simulink model "Teste_ModeloPV"  (R2017a)
settings: Solver=VariableStepAuto  StartTime=0.0  StopTime=10.0  MinStep=0.1  RelTol=1e-3
libraries: simulink x3, AvgModels x1
settings Model: Creator=lgalotto  LastModifiedBy=lgalotto

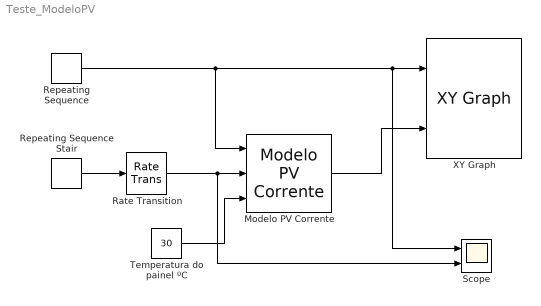
== system Teste_ModeloPV ==
  Modelo PV Corrente : AvgModels/Modelo PV Corrente  Ms=1  Mp=1  Ns=54  Voc=0.6093  Isc=8.21  Tr=273 + 25  Rs=0.005  Rp=7  a=3.18e-3  n=1.2  k=1.38e-23  q=1.60e-19  EG=1.1
      settings: SourceProductName=SimAverageModels
  Rate Transition : RateTransition  OutPortSampleTime=0.001
  Repeating Sequence : simulink/Sources/Repeating Sequence  rep_seq_t=[0 0.5 1]  rep_seq_y=[0 32 0]
  Repeating Sequence Stair : simulink/Sources/Repeating Sequence Stair  OutValues=[100 200 300 400 500 600 700 800 900 1000].'  tsamp=1  OutMin=[]  OutMax=[]  OutDataTypeStr=double  OutputDataTypeScalingMode=double  OutDataType=fixdt(0,8)  ConRadixGroup=Best Precision: Vector-wise  OutScaling=2^-12
  Scope : Scope  NumInputPorts=2
  Temperatura do painel ºC : Constant  Value=30
  XY Graph : simulink/Sinks/XY Graph  xmin=0  xmax=32  ymin=0  ymax=10  st=-1
  wires:
  Repeating Sequence Stair/1 -> Rate Transition/1
  Temperatura do painel ºC/1 -> Modelo PV Corrente/3
  Repeating Sequence/1 -> Modelo PV Corrente/1, Scope/1, XY Graph/1
  Modelo PV Corrente/1 -> XY Graph/2
  Rate Transition/1 -> Scope/2, Modelo PV Corrente/2
